simulink model "siso2"  (R2018a)
settings: Solver=VariableStepAuto  StartTime=0.0  StopTime=50.0  RelTol=1e-3
libraries: fuzblock x1
settings Model: Creator=root  LastModifiedBy=User
settings DebuggingCC: LibraryContextMissingDiagnostic=warning
settings SFSimCC: SimUseLocalCustomCode=on
settings RTWCC: RTWUseLocalCustomCode=on

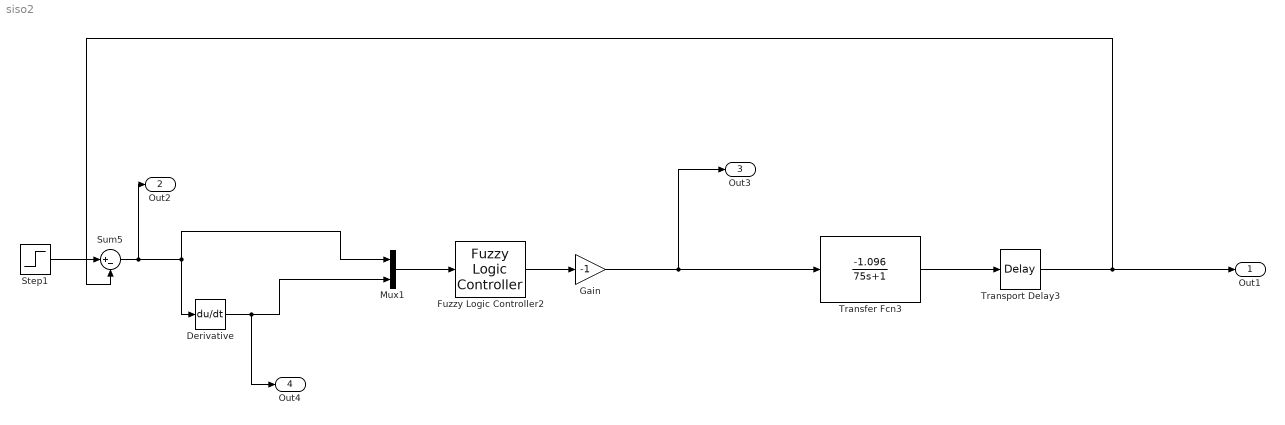
== system siso2 ==
  Derivative : Derivative
  Fuzzy Logic Controller2 : fuzblock/Fuzzy Logic  Controller  FIS=flc2  OutputSampleNumber=101  DataType=double  FuzzifiedInputs=off  RuleFiringStrengths=off  RuleOutputs=off  AggregatedOutputs=off  SimulateUsing=Interpreted execution  OutOfRangeInputValueMessage=warning  NoRuleFiredMessage=warning  EmptyOutputFuzzySetMessage=warning
  Gain : Gain  Gain=-1
  Mux1 : Mux  Inputs=2
  Step1 : Step  SampleTime=0
  Sum5 : Sum  Inputs=|+-
  Transfer Fcn3 : TransferFcn  Numerator=[-1.096]  Denominator=[75 1]
  Transport Delay3 : TransportDelay
  "Out1 " : Outport  SignalName=y2
  "Out2 " : Outport  Port=2  SignalName=Erro2
  Out3 : Outport  Port=3  SignalName=Control2
  Out4 : Outport  Port=4  SignalName=Derivada_erro2
  wires:
  Transfer Fcn3/1 -> Transport Delay3/1
  Fuzzy Logic Controller2/1 -> Gain/1
  Transport Delay3/1 -> Sum5/2, "Out1 "/1
  Step1/1 -> Sum5/1
  Sum5/1 -> Derivative/1, Mux1/1, "Out2 "/1
  Gain/1 -> Out3/1, Transfer Fcn3/1
  Mux1/1 -> Fuzzy Logic Controller2/1
  Derivative/1 -> Out4/1, Mux1/2
